simulink model "FinalSinScopes"  (R2023b)
settings: Solver=VariableStepAuto  StartTime=0.0  StopTime=10.0  RelTol=1e-3
values from neighbouring files (symbols this model uses):
  alfa_cu = 3.9E-3    (= 0.0039)    [Parametros.m]
  b_a = J_eq * n * omega_n    [MigracionPolosControladorExterno.m]    (also in Parametros.m = 1)
  b_eq = b_m + b_l/(r^2)    (= 2.19444444444e-05)    [Parametros.m]
  C_ts = 0.818    [Parametros.m]
  g = 9.80665    [Parametros.m]
  J_eq = J_m + J_l/(r^2)    [Parametros.m]
  k_l = m*l_cm + m_l(1)*l_l    [Parametros.m]
  K_sa = J_eq * n * omega_n^2    [MigracionPolosControladorExterno.m]    (also in Parametros.m = 1)
  K_sia = J_eq * omega_n^3    [MigracionPolosControladorExterno.m]    (also in Parametros.m = 1)
  Ke_int = 3.2768e10    (= 32768000000)    [Parametros.m]
  Ke_t = 6.4e3    (= 6400)    [Parametros.m]
  Ke_w = 1.024e7    (= 10240000)    [Parametros.m]
  L_d = 6.6E-3    (= 0.0066)    [Parametros.m]
  L_ls = 0.8E-3    (= 0.0008)    [Parametros.m]
  L_q = 5.8E-3    (= 0.0058)    [Parametros.m]
  lambda_m = 0.016    [Parametros.m]
  Mni_A = [0 -1; wn_mod^2 -2*zita_mod*wn_mod]    [Parametros.m]
  Mni_B = [1;0]    [Parametros.m]
  Mni_C = [0 1]    [Parametros.m]
  Mni_D = 0    [Parametros.m]
  P_p = 3    [Parametros.m]
  r = 120    [MigracionPolosControladorExterno.m]    (also in Parametros.m)
  R_tsamb = 146.7    [Parametros.m]
  Rs_ref = 1.02    [Parametros.m]
  Sni_A_iabc = [0 -1; wn_iabc^2 -2*wn_iabc*xi_iabc]    [Parametros.m]
  Sni_A_pos = [0 -1; wn_pos^2 -2*wn_pos*xi_pos]    [Parametros.m]
  Sni_A_T = -1/tau    (= -10)    [Parametros.m]
  Sni_B_iabc = [1; 0]    [Parametros.m]
  Sni_B_pos = [1; 0]    [Parametros.m]
  Sni_B_T = 1    [Parametros.m]
  Sni_C_iabc = [0 1]    [Parametros.m]
  Sni_C_pos = [0 1]    [Parametros.m]
  Sni_C_T = 1/tau    (= 10)    [Parametros.m]
  Sni_D_iabc = 0    [Parametros.m]
  Sni_D_pos = 0    [Parametros.m]
  Sni_D_T = 0    [Parametros.m]
  Tita_0 = 0    [Parametros.m]
  Ts = 1.25E-4    (= 0.000125)    [Parametros.m]
  Ts_0 = 20    [Parametros.m]
  Tsref = 20    [Parametros.m]
  V_slmax = 48    [Parametros.m]
settings Model: Creator=Home  LastModifiedBy=Home

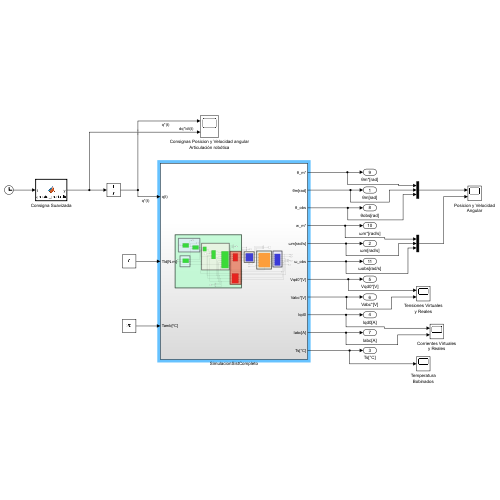
[thumbnail: Simulink's stored preview of the top-level diagram]
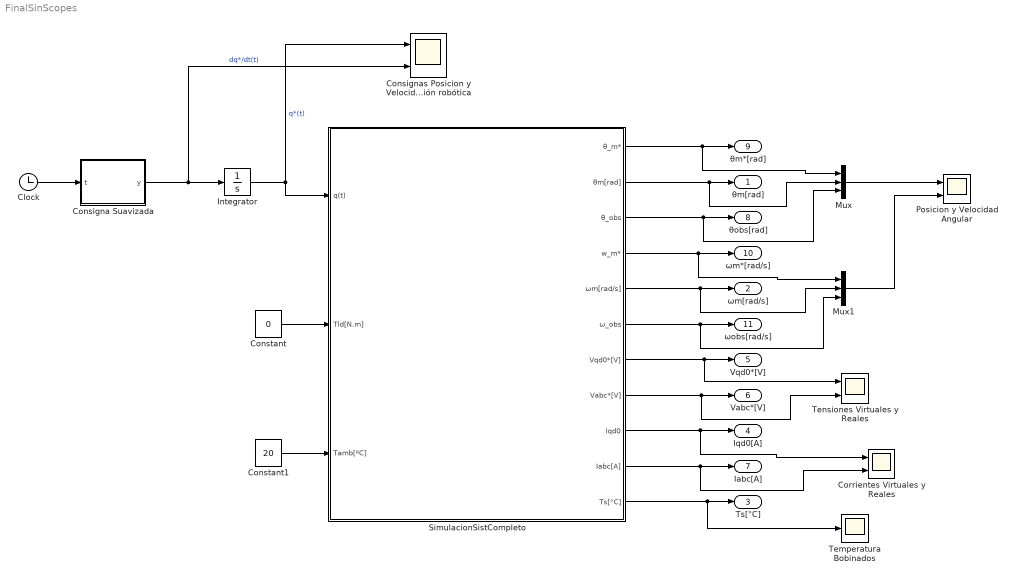
== system FinalSinScopes ==
  Clock : Clock
  Consigna Suavizada : MATLAB Function  TreatAsAtomicUnit=on
  Consignas Posicion y Velocidad angular Articulación robótica : Scope  NumInputPorts=2
  Constant : Constant  Value=0
  Constant1 : Constant  Value=20
  Corrientes Virtuales y Reales : Scope  NumInputPorts=2
  Integrator : Integrator
  Mux : Mux  Inputs=3
  Mux1 : Mux  Inputs=3
  Posicion y Velocidad Angular : Scope  NumInputPorts=2
  SimulacionSistCompleto : Subsystem
  Temperatura Bobinados : Scope
  Tensiones Virtuales y Reales : Scope  NumInputPorts=2
  θm[rad] : Outport
  ωm[rad/s] : Outport  Port=2
  Ts[°C] : Outport  Port=3
  Iqd0[A] : Outport  Port=4
  Vqd0*[V] : Outport  Port=5
  Vabc*[V] : Outport  Port=6
  Iabc[A] : Outport  Port=7
  θobs[rad] : Outport  Port=8
  θm*[rad] : Outport  Port=9
  ωm*[rad/s] : Outport  Port=10
  ωobs[rad/s] : Outport  Port=11
  wires:
  Integrator/1 -> Consignas Posicion y Velocidad angular Articulación robótica/1, SimulacionSistCompleto/1(q(t))  "q*(t)"
  SimulacionSistCompleto/2(θm[rad]) -> Mux/2, θm[rad]/1
  SimulacionSistCompleto/3(θ_obs) -> Mux/3, θobs[rad]/1
  Consigna Suavizada/1(y) -> Consignas Posicion y Velocidad angular Articulación robótica/2, Integrator/1  "dq*/dt(t)"
  Clock/1 -> Consigna Suavizada/1(t)
  Constant1/1 -> SimulacionSistCompleto/3(Tamb[ºC])
  SimulacionSistCompleto/1(θ_m*) -> Mux/1, θm*[rad]/1
  Constant/1 -> SimulacionSistCompleto/2(Tld[N.m])
  SimulacionSistCompleto/8(Vabc*[V]) -> Tensiones Virtuales y Reales/2, Vabc*[V]/1
  SimulacionSistCompleto/4(w_m*) -> Mux1/1, ωm*[rad/s]/1
  SimulacionSistCompleto/9(Iqd0) -> Corrientes Virtuales y Reales/1, Iqd0[A]/1
  SimulacionSistCompleto/5(ωm[rad/s]) -> Mux1/2, ωm[rad/s]/1
  SimulacionSistCompleto/10(Iabc[A]) -> Corrientes Virtuales y Reales/2, Iabc[A]/1
  SimulacionSistCompleto/11(Ts[°C]) -> Temperatura Bobinados/1, Ts[°C]/1
  SimulacionSistCompleto/7(Vqd0*[V]) -> Tensiones Virtuales y Reales/1, Vqd0*[V]/1
  SimulacionSistCompleto/6(ω_obs) -> Mux1/3, ωobs[rad/s]/1
  Mux/1 -> Posicion y Velocidad Angular/1
  Mux1/1 -> Posicion y Velocidad Angular/2

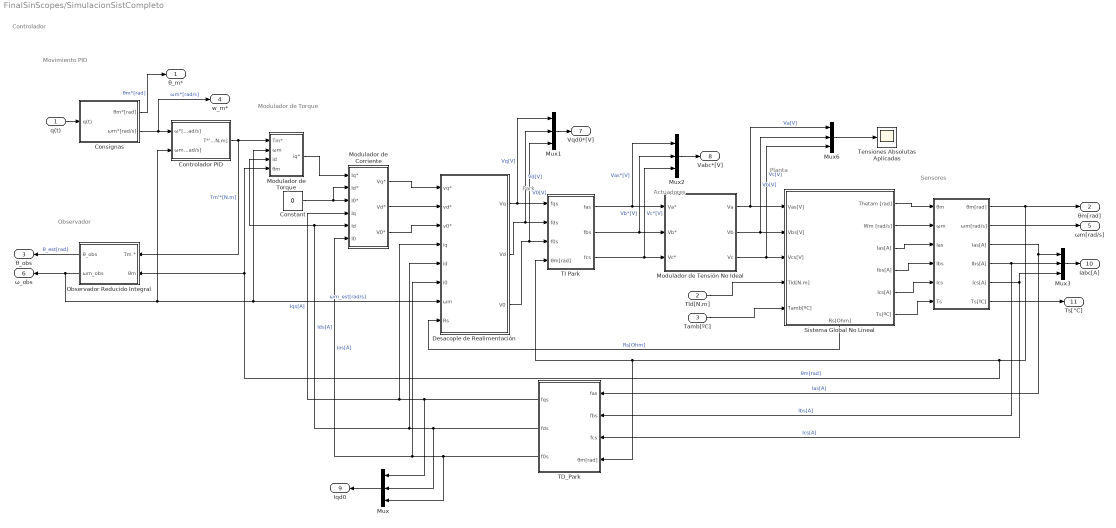
== system FinalSinScopes/SimulacionSistCompleto ==
  note: Sensores
  note: Park
  note: Observador
  note: Movimiento PID
  note: Modulador de Torque
  note: Controlador
  note: Actuadores
  note: Planta
  q(t) : Inport
  Tld[N.m] : Inport  Port=2
  Tamb[ºC] : Inport  Port=3
  " " : Subsystem
  Consignas : Subsystem
  Constant : Constant  Value=0
  Controlador PID : Subsystem
  Desacople de Realimentación : Subsystem
  Modulador de Corriente : Subsystem
  Modulador de Tensión No Ideal : Subsystem
  Modulador de Torque : Subsystem
  Mux{,1..3,6} (5 alike) : Mux  Inputs=3
  Observador Reducido Integral : Subsystem
  Sistema Global No Lineal : Subsystem
      settings: PortSchema="{\"entries\":[{\"content\":{\"sides\":[{\"content\":{\"connectorIds\":[\"In1\",\"In2\",\"In3\",\"In4\",\"In5\"]},\"type\":\"ConnectorPlacement.EquallySpacedRectSide\",\"uuid\":\"e69950d9-128a-479c-bb9c-058e9f1d4c4a\"},{\"content\":{\"connectorIds\":[\"Out1\",\"Out2\",\"Out3\",\"Out4\",\"Out5\",\"Out6\"],\"side\":\"RIGHT\"},\"type\":\"ConnectorPlacement.EquallySpacedRectSide\",\"uuid\":\"1754f544-d789-47dd-8fe5-32cce928f6e8\"},{\"content\":{\"side\":\"TOP\"},\"type\":\"ConnectorPlacement.EquallySpacedRectSide\",\"uuid\":\"429b420b-76ac-4d06-af5f-80d5ebf45ad3\"},{\"content\":{\"connectorIds\":[\"Out7\"],\"side\":\"BOTTOM\"},\"type\":\"ConnectorPlacement.EquallySpacedRectSide\",\"uuid\":\"85955431-78ef-4c8e-b012-5cf00baf8243\"}]},\"type\":\"ConnectorPlacement.EquallySpacedConnector\",\"uuid\":\"839c6553-6053-4832-bfe9-eda0736393b8\"}],\"packageUris\":[\"http://schema.mathworks.com/mf0/Connector/R2020b\"],\"version\":\"1.0\"}"
  TD_Park : Subsystem
  TI Park : Subsystem
  Tensiones Absolutas Aplicadas : Scope
  θ_m* : Outport
  θm[rad] : Outport  Port=2
  θ_obs : Outport  Port=3
  w_m* : Outport  Port=4
  ωm[rad/s] : Outport  Port=5
  ω_obs : Outport  Port=6
  Vqd0*[V] : Outport  Port=7
  Vabc*[V] : Outport  Port=8
  Iqd0 : Outport  Port=9
  Iabc[A] : Outport  Port=10
  Ts[°C] : Outport  Port=11
  wires:
  Consignas/2(ωm*[rad/s]) -> w_m*/1, Controlador PID/1(ω*[rad/s])  "ωm*[rad/s]"
  Modulador de Corriente/3(V0*) -> Desacople de Realimentación/3(v0*)
  Mux3/1 -> Iabc[A]/1
  TD_Park/2(fds) -> Modulador de Corriente/5(Id), Modulador de Torque/3(id), Desacople de Realimentación/5(id), Mux/2  "Ids[A]"
  TD_Park/1(fqs) -> Desacople de Realimentación/4(iq), Modulador de Corriente/4(Iq), Mux/1  "Iqs[A]"
  Modulador de Tensión No Ideal/3(Vc) -> Sistema Global No Lineal/3(Vcs[V]), Mux6/3  "Vc[V]"
  Modulador de Tensión No Ideal/1(Va) -> Sistema Global No Lineal/1(Vas[V]), Mux6/1  "Va[V]"
  Modulador de Torque/1(iq*) -> Modulador de Corriente/1(Iq*)
  TD_Park/3(f0s) -> Modulador de Corriente/6(I0), Desacople de Realimentación/6(i0), Mux/3  "Ios[A]"
  Modulador de Corriente/1(Vq*) -> Desacople de Realimentación/1(vq*)
  Desacople de Realimentación/2(Vd) -> Mux1/2, TI Park/2(fds)  "Vd[V]"
  Mux1/1 -> Vqd0*[V]/1
  Mux/1 -> Iqd0/1
  TI Park/1(fas) -> Modulador de Tensión No Ideal/1(Va*), Mux2/1  "Vas*[V]"
  TI Park/3(fcs) -> Modulador de Tensión No Ideal/3(Vc*), Mux2/3  "Vc*[V]"
  Tld[N.m]/1 -> Sistema Global No Lineal/4(Tld[N.m])
  Mux2/1 -> Vabc*[V]/1
  Tamb[ºC]/1 -> Sistema Global No Lineal/5(Tamb[ºC])
  Desacople de Realimentación/1(Vq) -> Mux1/1, TI Park/1(fqs)  "Vq[V]"
  Modulador de Corriente/2(Vd*) -> Desacople de Realimentación/2(vd*)
  Desacople de Realimentación/3(V0) -> Mux1/3, TI Park/3(f0s)  "V0[V]"
  q(t)/1 -> Consignas/1(q(t))
  Constant/1 -> Modulador de Corriente/3(I0*), Modulador de Corriente/2(Id*)
  TI Park/2(fbs) -> Modulador de Tensión No Ideal/2("Vb* "), Mux2/2  "Vb*[V]"
  Modulador de Tensión No Ideal/2(Vb) -> Sistema Global No Lineal/2(Vbs[V]), Mux6/2  "Vb[V]"
  Observador Reducido Integral/1(θ_obs) -> θ_obs/1  "θ_est[rad]"
  Controlador PID/1(T*'m[N.m]) -> Modulador de Torque/1(Tm*), Observador Reducido Integral/1(Tm *)  "Tm'*[N.m]"
  Observador Reducido Integral/2(ωm_obs) -> Desacople de Realimentación/7(ωm), Modulador de Torque/2(ωm), Controlador PID/2(ωm[rad/s]), ω_obs/1  "ωm_est[rad/s]"
  Consignas/1(θm*[rad]) -> θ_m*/1  "θm*[rad]"
  Sistema Global No Lineal/7(Rs[Ohm]) -> Desacople de Realimentación/8(Rs)  "Rs[Ohm]"
  Mux6/1 -> Tensiones Absolutas Aplicadas/1
  " "/3(Ias[A]) -> TD_Park/1(fas), Mux3/1  "Ias[A]"
  " "/5(Ics[A]) -> TD_Park/3(fcs), Mux3/3  "Ics[A]"
  " "/1(θm[rad]) -> θm[rad]/1, Observador Reducido Integral/2(θm), Modulador de Torque/4(θm), TD_Park/4(θm[rad]), TI Park/4(θm[rad])  "θm[rad]"
  " "/4(Ibs[A]) -> TD_Park/2(fbs), Mux3/2  "Ibs[A]"
  Sistema Global No Lineal/1(Thetam [rad]) -> " "/1(θm)
  Sistema Global No Lineal/2(Wm [rad/s]) -> " "/2(ωm)
  Sistema Global No Lineal/3(Ias[A]) -> " "/3(Ias)
  Sistema Global No Lineal/4(Ibs[A]) -> " "/4(Ibs)
  Sistema Global No Lineal/5(Ics[A]) -> " "/5(Ics)
  Sistema Global No Lineal/6(Ts[ºC]) -> " "/6(Ts)
  " "/2(ωm[rad/s]) -> ωm[rad/s]/1
  " "/6(Ts[ºC]) -> Ts[°C]/1

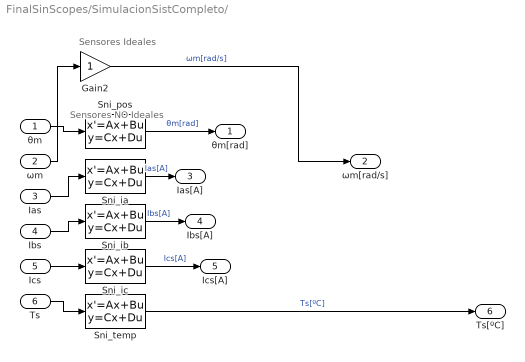
== system FinalSinScopes/SimulacionSistCompleto/  ==
  note: Sensores NO Ideales
  note: Sensores Ideales
  θm : Inport
  ωm : Inport  Port=2
  Ias : Inport  Port=3
  Ibs : Inport  Port=4
  Ics : Inport  Port=5
  Ts : Inport  Port=6
  Gain2 : Gain
  Sni_ia : StateSpace  A=Sni_A_iabc  B=Sni_B_iabc  C=Sni_C_iabc  D=Sni_D_iabc  InitialCondition=0
  Sni_ib : StateSpace  A=Sni_A_iabc  B=Sni_B_iabc  C=Sni_C_iabc  D=Sni_D_iabc  InitialCondition=0
  Sni_ic : StateSpace  A=Sni_A_iabc  B=Sni_B_iabc  C=Sni_C_iabc  D=Sni_D_iabc  InitialCondition=0
  Sni_pos : StateSpace  A=Sni_A_pos  B=Sni_B_pos  C=Sni_C_pos  D=Sni_D_pos  InitialCondition=0
  Sni_temp : StateSpace  A=Sni_A_T  B=Sni_B_T  C=Sni_C_T  D=Sni_D_T  InitialCondition=0
  θm[rad] : Outport
  ωm[rad/s] : Outport  Port=2
  Ias[A] : Outport  Port=3
  Ibs[A] : Outport  Port=4
  Ics[A] : Outport  Port=5
  Ts[ºC] : Outport  Port=6
  wires:
  Ics/1 -> Sni_ic/1
  Gain2/1 -> ωm[rad/s]/1  "ωm[rad/s]"
  Ibs/1 -> Sni_ib/1
  θm/1 -> Sni_pos/1
  Ts/1 -> Sni_temp/1
  Ias/1 -> Sni_ia/1
  Sni_temp/1 -> Ts[ºC]/1  "Ts[ºC]"
  Sni_pos/1 -> θm[rad]/1  "θm[rad]"
  ωm/1 -> Gain2/1
  Sni_ic/1 -> Ics[A]/1  "Ics[A]"
  Sni_ia/1 -> Ias[A]/1  "Ias[A]"
  Sni_ib/1 -> Ibs[A]/1  "Ibs[A]"

== system FinalSinScopes/SimulacionSistCompleto/Consignas ==
  q(t) : Inport
  Derivative : Derivative
  Gain : Gain  Gain=r
  θm*[rad] : Outport
  ωm*[rad/s] : Outport  Port=2
  wires:
  Derivative/1 -> ωm*[rad/s]/1
  Gain/1 -> θm*[rad]/1, Derivative/1
  q(t)/1 -> Gain/1

== system FinalSinScopes/SimulacionSistCompleto/Controlador PID ==
  ω*[rad/s] : Inport
  ωm[rad/s] : Inport  Port=2
  Gain : Gain  Gain=b_a
  Gain1 : Gain  Gain=K_sia
  Gain2 : Gain  Gain=K_sa
  Integracion Tustin : Subsystem
  Integracion Tustin1 : Subsystem
  Sum : Sum  Inputs=|+-
  Sum1 : Sum  Inputs=+++
  Zero-Order Hold : ZeroOrderHold  SampleTime=Ts
  Zero-Order Hold1 : ZeroOrderHold  SampleTime=Ts
  T*'m[N.m] : Outport
  wires:
  Sum1/1 -> Zero-Order Hold1/1
  Integracion Tustin1/1(y[k]) -> Gain1/1
  ω*[rad/s]/1 -> Sum/1
  Zero-Order Hold/1 -> Integracion Tustin/1(x[k]), Gain/1  "Ew"
  Gain2/1 -> Sum1/2
  Integracion Tustin/1(y[k]) -> Integracion Tustin1/1(x[k]), Gain2/1  "Eθ"
  ωm[rad/s]/1 -> Sum/2
  Gain/1 -> Sum1/3
  Gain1/1 -> Sum1/1
  Sum/1 -> Zero-Order Hold/1  "Ew"
  Zero-Order Hold1/1 -> T*'m[N.m]/1

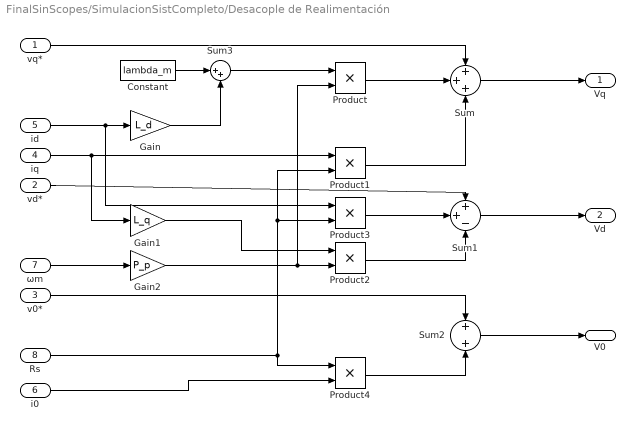
== system FinalSinScopes/SimulacionSistCompleto/Desacople de Realimentación ==
  vq* : Inport
  vd* : Inport  Port=2
  v0* : Inport  Port=3
  iq : Inport  Port=4
  id : Inport  Port=5
  i0 : Inport  Port=6
  ωm : Inport  Port=7
  Rs : Inport  Port=8
  Constant : Constant  Value=lambda_m
  Gain : Gain  Gain=L_d
  Gain1 : Gain  Gain=L_q
  Gain2 : Gain  Gain=P_p
  Product{,1..4} (5 alike) : Product
  Sum : Sum  Inputs=+++
  Sum1 : Sum  Inputs=++-
  Sum2 : Sum  Inputs=+|+
  Sum3 : Sum  Inputs=|++
  Vq : Outport
  Vd : Outport  Port=2
  V0 : Outport  Port=3
  wires:
  ωm/1 -> Gain2/1
  Sum/1 -> Vq/1
  Rs/1 -> Product4/1, Product1/2, Product3/2
  Gain/1 -> Sum3/2
  Product/1 -> Sum/2
  Sum2/1 -> V0/1
  Product4/1 -> Sum2/2
  Sum3/1 -> Product/1
  id/1 -> Product3/1, Gain/1
  vq*/1 -> Sum/1
  i0/1 -> Product4/2
  iq/1 -> Product1/1, Gain1/1
  Product2/1 -> Sum1/3
  Constant/1 -> Sum3/1
  v0*/1 -> Sum2/1
  Product1/1 -> Sum/3
  Gain2/1 -> Product/2, Product2/2
  vd*/1 -> Sum1/1
  Gain1/1 -> Product2/1
  Sum1/1 -> Vd/1
  Product3/1 -> Sum1/2

== system FinalSinScopes/SimulacionSistCompleto/Modulador de Corriente ==
  Iq* : Inport
  Id* : Inport  Port=2
  I0* : Inport  Port=3
  Iq : Inport  Port=4
  Id : Inport  Port=5
  I0 : Inport  Port=6
  Gain : Gain  Gain=5000*L_q
  Gain1 : Gain  Gain=5000*L_d
  Gain2 : Gain  Gain=5000*L_ls
  Sum : Sum  Inputs=|+-
  Sum1 : Sum  Inputs=|+-
  Sum2 : Sum  Inputs=|+-
  Vq* : Outport
  Vd* : Outport  Port=2
  V0* : Outport  Port=3
  wires:
  Gain2/1 -> V0*/1
  Sum/1 -> Gain/1
  Sum1/1 -> Gain1/1
  Gain/1 -> Vq*/1
  Iq/1 -> Sum/2
  I0*/1 -> Sum2/1
  Iq*/1 -> Sum/1
  Id/1 -> Sum1/2
  Sum2/1 -> Gain2/1
  Id*/1 -> Sum1/1
  Gain1/1 -> Vd*/1
  I0/1 -> Sum2/2

== system FinalSinScopes/SimulacionSistCompleto/Modulador de Tensión No Ideal ==
  Va* : Inport
  "Vb* " : Inport  Port=2
  Vc* : Inport  Port=3
  Saturation : Saturate  UpperLimit=sqrt(2/3)*V_slmax  LowerLimit=-sqrt(2/3)*V_slmax
  Saturation1 : Saturate  UpperLimit=sqrt(2/3)*V_slmax  LowerLimit=-sqrt(2/3)*V_slmax
  Saturation2 : Saturate  UpperLimit=sqrt(2/3)*V_slmax  LowerLimit=-sqrt(2/3)*V_slmax
  State-Space : StateSpace  A=Mni_A  B=Mni_B  C=Mni_C  D=Mni_D  InitialCondition=0
  State-Space1 : StateSpace  A=Mni_A  B=Mni_B  C=Mni_C  D=Mni_D  InitialCondition=0
  State-Space2 : StateSpace  A=Mni_A  B=Mni_B  C=Mni_C  D=Mni_D  InitialCondition=0
  Va : Outport
  Vb : Outport  Port=2
  Vc : Outport  Port=3
  wires:
  Vc*/1 -> State-Space2/1
  "Vb* "/1 -> State-Space1/1
  State-Space/1 -> Saturation/1
  Va*/1 -> State-Space/1
  State-Space1/1 -> Saturation1/1
  State-Space2/1 -> Saturation2/1
  Saturation/1 -> Va/1
  Saturation1/1 -> Vb/1
  Saturation2/1 -> Vc/1

== system FinalSinScopes/SimulacionSistCompleto/Modulador de Torque ==
  Tm* : Inport
  ωm : Inport  Port=2
  id : Inport  Port=3
  θm : Inport  Port=4
  Constant : Constant  Value=L_d
  Constant1 : Constant  Value=L_q
  Constant2 : Constant  Value=lambda_m
  Divide : Product  Inputs=*/
  Gain : Gain  Gain=b_eq
  Gain1 : Gain  Gain=3/2*P_p
  Gain2 : Gain  Gain=1/r
  Gain3 : Gain  Gain=k_l*g/r
  Product : Product
  Sin : Trigonometry
  Sum : Sum  Inputs=+++
  Sum1 : Sum  Inputs=|+-
  Sum2 : Sum  Inputs=|++
  iq* : Outport
  wires:
  Constant2/1 -> Sum2/2
  ωm/1 -> Gain/1
  Sum1/1 -> Product/2
  Gain3/1 -> Sum/1
  θm/1 -> Gain2/1  "θm"
  Sum2/1 -> Gain1/1
  Constant/1 -> Sum1/1
  Gain1/1 -> Divide/2
  Divide/1 -> iq*/1
  Product/1 -> Sum2/1
  Gain/1 -> Sum/3
  Constant1/1 -> Sum1/2
  Sin/1 -> Gain3/1
  Gain2/1 -> Sin/1
  Sum/1 -> Divide/1
  id/1 -> Product/1
  Tm*/1 -> Sum/2

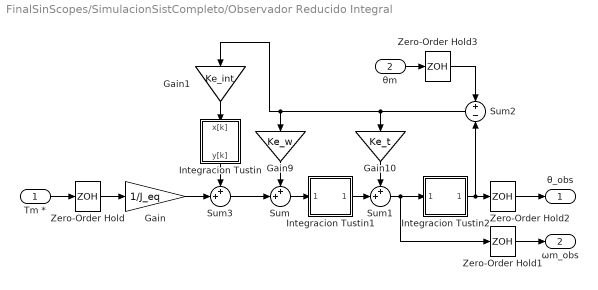
== system FinalSinScopes/SimulacionSistCompleto/Observador Reducido Integral ==
  Tm * : Inport
  θm : Inport  Port=2
  Gain : Gain  Gain=1/J_eq
  Gain1 : Gain  Gain=Ke_int
  Gain10 : Gain  Gain=Ke_t
  Gain9 : Gain  Gain=Ke_w
  Integracion Tustin : Subsystem
  Integracion Tustin1 : Subsystem
  Integracion Tustin2 : Subsystem
  Sum : Sum  Inputs=++|
  Sum1 : Sum  Inputs=++|
  Sum2 : Sum  Inputs=+|-
  Sum3 : Sum  Inputs=++|
  Zero-Order Hold{,1..3} (4 alike) : ZeroOrderHold  SampleTime=-1
  θ_obs : Outport
  ωm_obs : Outport  Port=2
  wires:
  Gain10/1 -> Sum1/1
  Sum2/1 -> Gain1/1, Gain9/1, Gain10/1
  Integracion Tustin2/1(y[k]) -> Zero-Order Hold2/1, Sum2/2
  Tm */1 -> Zero-Order Hold/1
  θm/1 -> Zero-Order Hold3/1
  Sum1/1 -> Integracion Tustin2/1(x[k]), Zero-Order Hold1/1
  Integracion Tustin1/1(y[k]) -> Sum1/2
  Sum/1 -> Integracion Tustin1/1(x[k])
  Gain/1 -> Sum3/2
  Gain9/1 -> Sum/1
  Sum3/1 -> Sum/2
  Gain1/1 -> Integracion Tustin/1(x[k])
  Integracion Tustin/1(y[k]) -> Sum3/1
  Zero-Order Hold/1 -> Gain/1
  Zero-Order Hold1/1 -> ωm_obs/1
  Zero-Order Hold2/1 -> θ_obs/1
  Zero-Order Hold3/1 -> Sum2/1

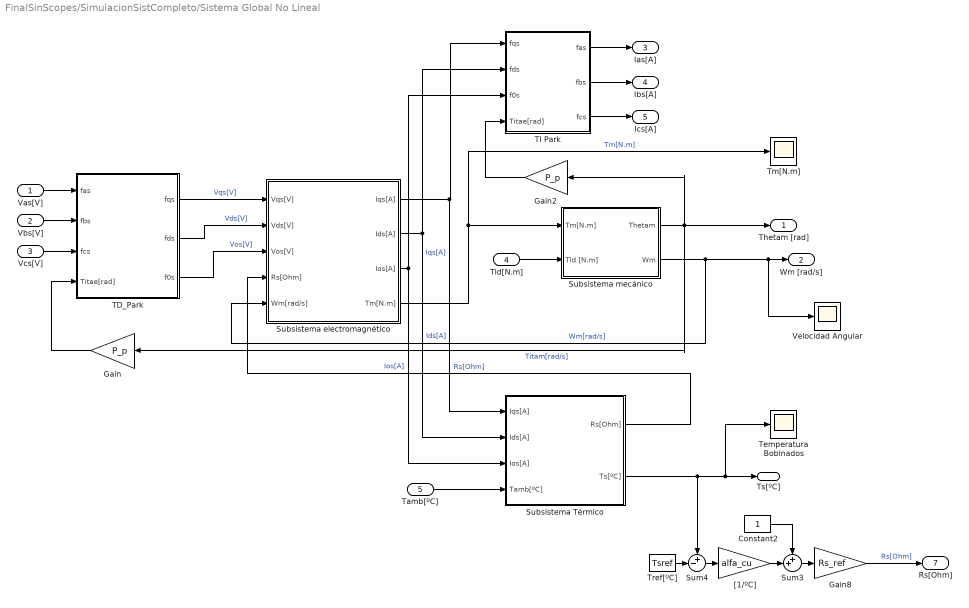
== system FinalSinScopes/SimulacionSistCompleto/Sistema Global No Lineal ==
  Vas[V] : Inport
  Vbs[V] : Inport  Port=2
  Vcs[V] : Inport  Port=3
  Tld[N.m] : Inport  Port=4
  Tamb[ºC] : Inport  Port=5
  Constant2 : Constant
  Gain : Gain  Gain=P_p
  Gain2 : Gain  Gain=P_p
  Gain8 : Gain  Gain=Rs_ref
  Subsistema Térmico : Subsystem
  Subsistema electromagnético : Subsystem
  Subsistema mecánico : Subsystem
  Sum3 : Sum  Inputs=++|
  Sum4 : Sum  Inputs=+-|
  TD_Park : Subsystem
  TI Park : Subsystem
  Temperatura Bobinados : Scope
  Tm[N.m] : Scope
  Tref[ºC] : Constant  Value=Tsref
  Velocidad Angular : Scope
  "[1/ºC]" : Gain  Gain=alfa_cu
  Thetam [rad] : Outport
  Wm [rad/s] : Outport  Port=2
  Ias[A] : Outport  Port=3
  Ibs[A] : Outport  Port=4
  Ics[A] : Outport  Port=5
  Ts[ºC] : Outport  Port=6
  Rs[Ohm] : Outport  Port=7
  wires:
  Subsistema electromagnético/3(Ios[A]) -> Subsistema Térmico/3(Ios[A]), TI Park/3(f0s)  "Ios[A]"
  Subsistema mecánico/2(Wm) -> Velocidad Angular/1, Wm [rad/s]/1, Subsistema electromagnético/5(Wm[rad/s])  "Wm[rad/s]"
  TD_Park/3(f0s) -> Subsistema electromagnético/3(Vos[V])  "Vos[V]"
  Gain/1 -> TD_Park/4(Titae[rad])
  Subsistema Térmico/1(Rs[Ohm]) -> Subsistema electromagnético/4(Rs[Ohm])  "Rs[Ohm]"
  TD_Park/1(fqs) -> Subsistema electromagnético/1(Vqs[V])  "Vqs[V]"
  Vbs[V]/1 -> TD_Park/2(fbs)
  Vcs[V]/1 -> TD_Park/3(fcs)
  Subsistema electromagnético/1(Iqs[A]) -> Subsistema Térmico/1(Iqs[A]), TI Park/1(fqs)  "Iqs[A]"
  Subsistema electromagnético/4(Tm[N.m]) -> Tm[N.m]/1, Subsistema mecánico/1(Tm[N.m])  "Tm[N.m]"
  Subsistema mecánico/1(Thetam) -> Thetam [rad]/1, Gain2/1, Gain/1  "Titam[rad/s]"
  Tamb[ºC]/1 -> Subsistema Térmico/4(Tamb[ºC])
  Vas[V]/1 -> TD_Park/1(fas)
  TD_Park/2(fds) -> Subsistema electromagnético/2(Vds[V])  "Vds[V]"
  TI Park/2(fbs) -> Ibs[A]/1
  Subsistema electromagnético/2(Ids[A]) -> TI Park/2(fds), Subsistema Térmico/2(Ids[A])  "Ids[A]"
  Gain2/1 -> TI Park/4(Titae[rad])
  TI Park/1(fas) -> Ias[A]/1
  Subsistema Térmico/2(Ts[ºC]) -> Sum4/1, Temperatura Bobinados/1, Ts[ºC]/1
  Tld[N.m]/1 -> Subsistema mecánico/2(Tld [N.m])
  TI Park/3(fcs) -> Ics[A]/1
  "[1/ºC]"/1 -> Sum3/2
  Sum3/1 -> Gain8/1
  Tref[ºC]/1 -> Sum4/2
  Constant2/1 -> Sum3/1
  Sum4/1 -> "[1/ºC]"/1
  Gain8/1 -> Rs[Ohm]/1  "Rs[Ohm]"

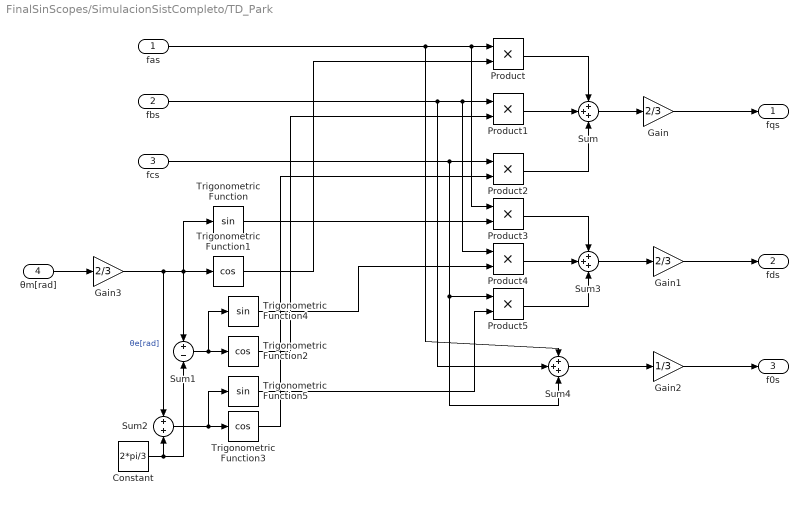
== system FinalSinScopes/SimulacionSistCompleto/TD_Park ==
  fas : Inport
  fbs : Inport  Port=2
  fcs : Inport  Port=3
  θm[rad] : Inport  Port=4
  Constant : Constant  Value=2*pi/3
  Gain : Gain  Gain=2/3
  Gain1 : Gain  Gain=2/3
  Gain2 : Gain  Gain=1/3
  Gain3 : Gain  Gain=2/3
  Product{,1..5} (6 alike) : Product
  Sum : Sum  Inputs=+++
  Sum1 : Sum  Inputs=+-
  Sum2 : Sum
  Sum3 : Sum  Inputs=+++
  Sum4 : Sum  Inputs=+++
  Trigonometric Function : Trigonometry
  Trigonometric Function1 : Trigonometry  Operator=cos
  Trigonometric Function2 : Trigonometry  Operator=cos
  Trigonometric Function3 : Trigonometry  Operator=cos
  Trigonometric Function4 : Trigonometry
  Trigonometric Function5 : Trigonometry
  fqs : Outport
  fds : Outport  Port=2
  f0s : Outport  Port=3
  wires:
  fas/1 -> Sum4/1, Product3/1, Product/1
  Trigonometric Function3/1 -> Product2/2
  Sum1/1 -> Trigonometric Function4/1, Trigonometric Function2/1
  Constant/1 -> Sum2/2, Sum1/2
  Trigonometric Function1/1 -> Product/2
  fcs/1 -> Product5/1, Sum4/3, Product2/1
  Product5/1 -> Sum3/3
  Product/1 -> Sum/1
  Product3/1 -> Sum3/1
  Product1/1 -> Sum/2
  Trigonometric Function/1 -> Product3/2
  Sum2/1 -> Trigonometric Function5/1, Trigonometric Function3/1
  Trigonometric Function5/1 -> Product5/2
  Sum4/1 -> Gain2/1
  fbs/1 -> Sum4/2, Product4/1, Product1/1
  Product2/1 -> Sum/3
  Gain/1 -> fqs/1
  Trigonometric Function4/1 -> Product4/2
  Product4/1 -> Sum3/2
  Trigonometric Function2/1 -> Product1/2
  Gain2/1 -> f0s/1
  Sum/1 -> Gain/1
  Gain1/1 -> fds/1
  Sum3/1 -> Gain1/1
  θm[rad]/1 -> Gain3/1
  Gain3/1 -> Sum2/1, Trigonometric Function/1, Sum1/1, Trigonometric Function1/1  "θe[rad]"

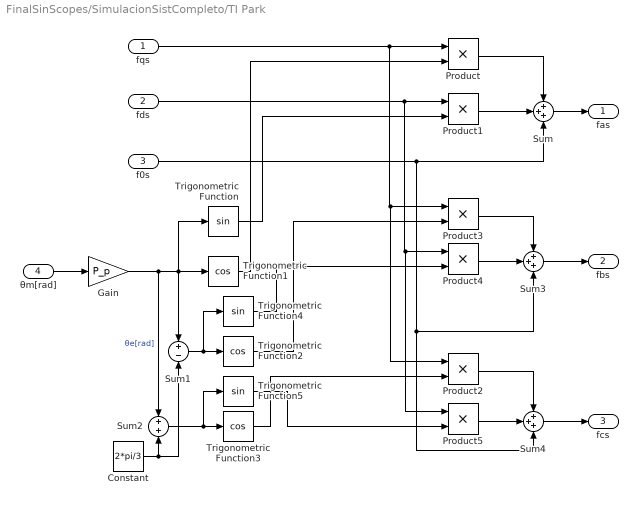
== system FinalSinScopes/SimulacionSistCompleto/TI Park ==
  fqs : Inport
  fds : Inport  Port=2
  f0s : Inport  Port=3
  θm[rad] : Inport  Port=4
  Constant : Constant  Value=2*pi/3
  Gain : Gain  Gain=P_p
  Product{,1..5} (6 alike) : Product
  Sum : Sum  Inputs=+++
  Sum1 : Sum  Inputs=+-
  Sum2 : Sum
  Sum3 : Sum  Inputs=+++
  Sum4 : Sum  Inputs=+++
  Trigonometric Function : Trigonometry
  Trigonometric Function1 : Trigonometry  Operator=cos
  Trigonometric Function2 : Trigonometry  Operator=cos
  Trigonometric Function3 : Trigonometry  Operator=cos
  Trigonometric Function4 : Trigonometry
  Trigonometric Function5 : Trigonometry
  fas : Outport
  fbs : Outport  Port=2
  fcs : Outport  Port=3
  wires:
  Constant/1 -> Sum2/2, Sum1/2
  Product1/1 -> Sum/2
  Trigonometric Function2/1 -> Product3/2
  Trigonometric Function5/1 -> Product5/2
  fds/1 -> Product1/1, Product5/1, Product4/1
  f0s/1 -> Sum/3, Sum3/3, Sum4/3
  Product3/1 -> Sum3/1
  fqs/1 -> Product/1, Product2/1, Product3/1
  Product2/1 -> Sum4/1
  Trigonometric Function1/1 -> Product/2
  Product/1 -> Sum/1
  Sum2/1 -> Trigonometric Function5/1, Trigonometric Function3/1
  Sum1/1 -> Trigonometric Function4/1, Trigonometric Function2/1
  Trigonometric Function/1 -> Product1/2
  Product4/1 -> Sum3/2
  Sum/1 -> fas/1
  Trigonometric Function3/1 -> Product2/2
  Product5/1 -> Sum4/2
  Trigonometric Function4/1 -> Product4/2
  Sum3/1 -> fbs/1
  Sum4/1 -> fcs/1
  θm[rad]/1 -> Gain/1
  Gain/1 -> Sum2/1, Trigonometric Function/1, Sum1/1, Trigonometric Function1/1  "θe[rad]"

== system FinalSinScopes/SimulacionSistCompleto/Controlador PID/Integracion Tustin ==
  x[k] : Inport
  Delay : Delay  DelayLength=1
  Delay1 : Delay  DelayLength=1
  Gain3 : Gain  Gain=Ts/2
  Sum2 : Sum  Inputs=|++
  Sum3 : Sum  Inputs=|++
  y[k] : Outport
  wires:
  x[k]/1 -> Delay/1, Sum3/1
  Sum2/1 -> y[k]/1, Delay1/1
  Delay1/1 -> Sum2/2
  Sum3/1 -> Gain3/1
  Delay/1 -> Sum3/2
  Gain3/1 -> Sum2/1

== system FinalSinScopes/SimulacionSistCompleto/Controlador PID/Integracion Tustin1 ==
  x[k] : Inport
  Delay : Delay  DelayLength=1
  Delay1 : Delay  DelayLength=1
  Gain3 : Gain  Gain=Ts/2
  Sum2 : Sum  Inputs=|++
  Sum3 : Sum  Inputs=|++
  y[k] : Outport
  wires:
  x[k]/1 -> Delay/1, Sum3/1
  Sum2/1 -> y[k]/1, Delay1/1
  Delay1/1 -> Sum2/2
  Sum3/1 -> Gain3/1
  Delay/1 -> Sum3/2
  Gain3/1 -> Sum2/1

== system FinalSinScopes/SimulacionSistCompleto/Observador Reducido Integral/Integracion Tustin ==
  x[k] : Inport
  Delay : Delay  DelayLength=1
  Delay1 : Delay  DelayLength=1
  Gain3 : Gain  Gain=Ts/2
  Sum2 : Sum  Inputs=|++
  Sum3 : Sum  Inputs=|++
  y[k] : Outport
  wires:
  x[k]/1 -> Delay/1, Sum3/1
  Sum2/1 -> y[k]/1, Delay1/1
  Delay1/1 -> Sum2/2
  Sum3/1 -> Gain3/1
  Delay/1 -> Sum3/2
  Gain3/1 -> Sum2/1

== system FinalSinScopes/SimulacionSistCompleto/Observador Reducido Integral/Integracion Tustin1 ==
  x[k] : Inport
  Delay : Delay  DelayLength=1
  Delay1 : Delay  DelayLength=1
  Gain3 : Gain  Gain=Ts/2
  Sum2 : Sum  Inputs=|++
  Sum3 : Sum  Inputs=|++
  y[k] : Outport
  wires:
  x[k]/1 -> Delay/1, Sum3/1
  Sum2/1 -> y[k]/1, Delay1/1
  Delay1/1 -> Sum2/2
  Sum3/1 -> Gain3/1
  Delay/1 -> Sum3/2
  Gain3/1 -> Sum2/1

== system FinalSinScopes/SimulacionSistCompleto/Observador Reducido Integral/Integracion Tustin2 ==
  x[k] : Inport
  Delay : Delay  DelayLength=1
  Delay1 : Delay  DelayLength=1
  Gain3 : Gain  Gain=Ts/2
  Sum2 : Sum  Inputs=|++
  Sum3 : Sum  Inputs=|++
  y[k] : Outport
  wires:
  x[k]/1 -> Delay/1, Sum3/1
  Sum2/1 -> y[k]/1, Delay1/1
  Delay1/1 -> Sum2/2
  Sum3/1 -> Gain3/1
  Delay/1 -> Sum3/2
  Gain3/1 -> Sum2/1

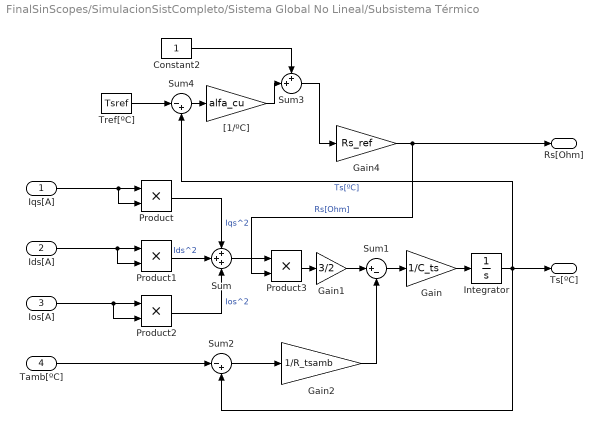
== system FinalSinScopes/SimulacionSistCompleto/Sistema Global No Lineal/Subsistema Térmico ==
  Iqs[A] : Inport
  Ids[A] : Inport  Port=2
  Ios[A] : Inport  Port=3
  Tamb[ºC] : Inport  Port=4
  Constant2 : Constant
  Gain : Gain  Gain=1/C_ts
  Gain1 : Gain  Gain=3/2
  Gain2 : Gain  Gain=1/R_tsamb
  Gain4 : Gain  Gain=Rs_ref
  Integrator : Integrator  InitialCondition=Ts_0
  Product{,1..3} (4 alike) : Product
  Sum : Sum  Inputs=+++
  Sum1 : Sum  Inputs=|+-
  Sum2 : Sum  Inputs=|-+
  Sum3 : Sum  Inputs=++|
  Sum4 : Sum  Inputs=|-+
  Tref[ºC] : Constant  Value=Tsref
  "[1/ºC]" : Gain  Gain=alfa_cu
  Rs[Ohm] : Outport
  Ts[ºC] : Outport  Port=2
  wires:
  Sum3/1 -> Gain4/1
  Gain/1 -> Integrator/1
  Product1/1 -> Sum/2  "Ids^2"
  Product/1 -> Sum/1  "Iqs^2"
  Sum/1 -> Product3/1
  Iqs[A]/1 -> Product/2, Product/1
  Ids[A]/1 -> Product1/2, Product1/1
  Product2/1 -> Sum/3  "Ios^2"
  Sum4/1 -> "[1/ºC]"/1
  Tamb[ºC]/1 -> Sum2/1
  Sum1/1 -> Gain/1
  Sum2/1 -> Gain2/1
  Gain4/1 -> Rs[Ohm]/1, Product3/2  "Rs[Ohm]"
  Gain1/1 -> Sum1/1
  Ios[A]/1 -> Product2/2, Product2/1
  Constant2/1 -> Sum3/1
  Tref[ºC]/1 -> Sum4/1
  Product3/1 -> Gain1/1
  "[1/ºC]"/1 -> Sum3/2
  Gain2/1 -> Sum1/2
  Integrator/1 -> Ts[ºC]/1, Sum2/2, Sum4/2  "Ts[ºC]"

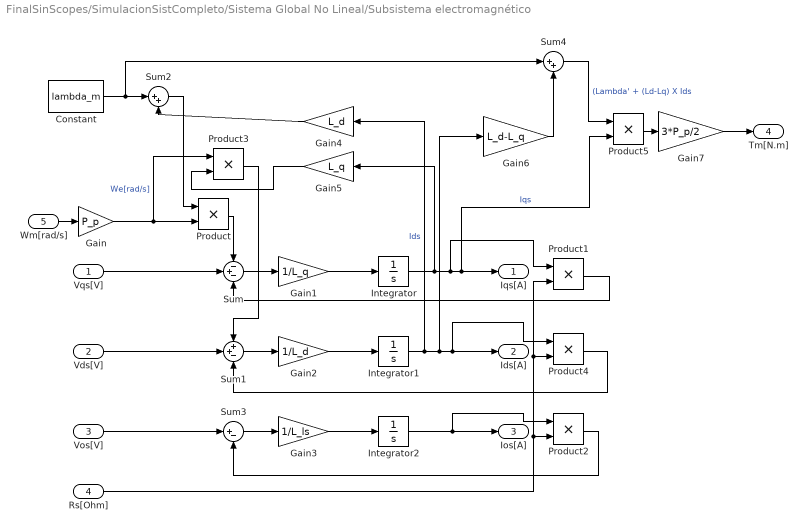
== system FinalSinScopes/SimulacionSistCompleto/Sistema Global No Lineal/Subsistema electromagnético ==
  Vqs[V] : Inport
  Vds[V] : Inport  Port=2
  Vos[V] : Inport  Port=3
  Rs[Ohm] : Inport  Port=4
  Wm[rad/s] : Inport  Port=5
  Constant : Constant  Value=lambda_m
  Gain : Gain  Gain=P_p
  Gain1 : Gain  Gain=1/L_q
  Gain2 : Gain  Gain=1/L_d
  Gain3 : Gain  Gain=1/L_ls
  Gain4 : Gain  Gain=L_d
  Gain5 : Gain  Gain=L_q
  Gain6 : Gain  Gain=L_d-L_q
  Gain7 : Gain  Gain=3*P_p/2
  Integrator : Integrator
  Integrator1 : Integrator  InitialCondition=-0.5
  Integrator2 : Integrator
  Product{,1..5} (6 alike) : Product
  Sum : Sum  Inputs=-+-
  Sum1 : Sum  Inputs=++-
  Sum2 : Sum  Inputs=|++
  Sum3 : Sum  Inputs=|+-
  Sum4 : Sum  Inputs=|++
  Iqs[A] : Outport
  Ids[A] : Outport  Port=2
  Ios[A] : Outport  Port=3
  Tm[N.m] : Outport  Port=4
  wires:
  Product3/1 -> Sum1/1
  Gain5/1 -> Product3/2
  Vos[V]/1 -> Sum3/1
  Sum1/1 -> Gain2/1
  Integrator/1 -> Gain5/1, Product1/1, Iqs[A]/1, Product5/2  "Iqs"
  Integrator2/1 -> Ios[A]/1, Product2/1
  Rs[Ohm]/1 -> Product4/2, Product1/2, Product2/2
  Product1/1 -> Sum/3
  Sum/1 -> Gain1/1
  Sum4/1 -> Product5/1  "(Lambda' + (Ld-Lq) X Ids"
  Integrator1/1 -> Gain6/1, Ids[A]/1, Product4/1, Gain4/1  "Ids"
  Gain/1 -> Product/2, Product3/1  "We[rad/s]"
  Sum3/1 -> Gain3/1
  Gain6/1 -> Sum4/2
  Wm[rad/s]/1 -> Gain/1
  Gain7/1 -> Tm[N.m]/1
  Product5/1 -> Gain7/1
  Vqs[V]/1 -> Sum/2
  Gain2/1 -> Integrator1/1
  Product/1 -> Sum/1
  Constant/1 -> Sum4/1, Sum2/1
  Sum2/1 -> Product/1
  Vds[V]/1 -> Sum1/2
  Gain4/1 -> Sum2/2
  Product4/1 -> Sum1/3
  Product2/1 -> Sum3/2
  Gain1/1 -> Integrator/1
  Gain3/1 -> Integrator2/1

== system FinalSinScopes/SimulacionSistCompleto/Sistema Global No Lineal/Subsistema mecánico ==
  note: beq [N.m/{rad/s}]
  note: 1/Jeq [kg.m^2]
  Tm[N.m] : Inport
  Tld [N.m] : Inport  Port=2
  Gain : Gain  Gain=1/J_eq
  Gain1 : Gain  Gain=b_eq
  Gain2 : Gain  Gain=g*k_l/r
  Gain3 : Gain  Gain=1/r
  Gain4 : Gain  Gain=1/r
  Integrator : Integrator
  Integrator1 : Integrator  InitialCondition=Tita_0
  Perturbacion TL : Scope
  Sum1 : Sum  Inputs=-+-
  Sum2 : Sum  Inputs=|++
  TorqueEq : Scope
  TorqueFriccion : Scope
  Trigonometric Function : Trigonometry
  XY Graph : Record  FileSettingsInternal="{\"entries\":[{\"content\":{\"excelSettings\":{\"content\":{},\"type\":\"Streamout.ExcelSettings\"}},\"type\":\"Streamout.FileSettingStorage\",\"uuid\":\"\"}],\"packageUris\":[\"http:\\/\\/schema.mathworks.com\\/mf0\\/streamout_blocks\\/R2020a\"],\"version\":\"1.0\"}"  Layout=[1 1]  SignalsInternal="{\"entries\":[{\"content\":{\"signals\":[{\"content\":{\"blockPath\":[],\"dimensions\":[1],\"domain\":\"\",\"lineColor\":\"#ff6929\",\"port\":1,\"signalID\":14343,\"signalName\":\"Wm[rad\\/s]\"},\"type\":\"RecordBlkView.Signal\",\"uuid\":\"\"},{\"content\":{\"blockPath\":[],\"dimensions\":[1],\"domain\":\"\",\"lineColor\":\"#b746ff\",\"port\":2,\"signalID\":14346,\"signalName\":\"Tm[N.m]\"},\"type\":\"RecordBlkView.Signal\",\"uuid\":\"\"}]},\"type\":\"RecordBlkView.InputSignals\",\"uuid\":\"\"}],\"packageUris\":[\"http:\\/\\/schema.mathworks.com\\/mf0\\/streamout_blocks\\/R2020a\"],\"version\":\"1.0\"}"  VisualizationBindings="{\"xyplotplugin\":{\"info\":[{\"series\":[],\"subplotID\":1}]}}"  CompatibilityTag=XY
  Thetam : Outport
  Wm : Outport  Port=2
  wires:
  Tld [N.m]/1 -> Gain4/1
  Gain3/1 -> Trigonometric Function/1  "Thetal[rad]"
  Tm[N.m]/1 -> XY Graph/2, Sum1/2  "Tm[N.m]"
  Integrator/1 -> XY Graph/1, Wm/1, Gain1/1, Integrator1/1  "Wm[rad/s]"
  Integrator1/1 -> Thetam/1, Gain3/1  "Thetam[rad]"
  Trigonometric Function/1 -> Gain2/1
  Gain1/1 -> TorqueFriccion/1, Sum1/3
  Gain/1 -> Integrator/1  "dWm/dt[rad/s^2]"
  Sum1/1 -> TorqueEq/1, Gain/1
  Gain4/1 -> Sum2/1
  Gain2/1 -> Sum2/2
  Sum2/1 -> Perturbacion TL/1, Sum1/1

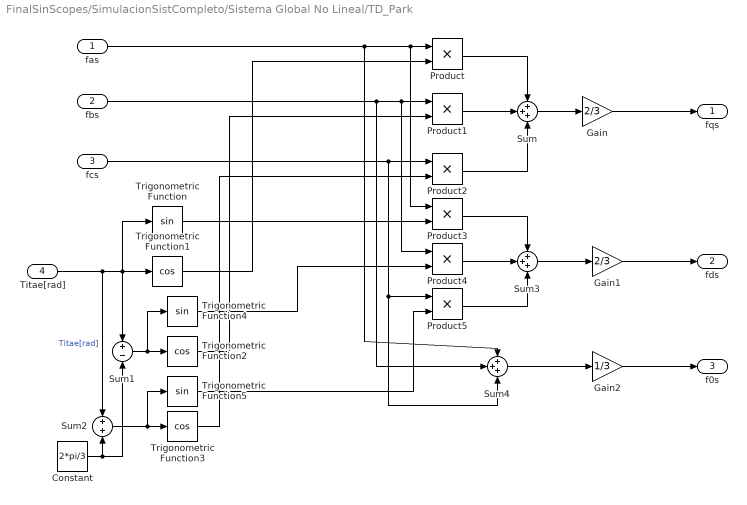
== system FinalSinScopes/SimulacionSistCompleto/Sistema Global No Lineal/TD_Park ==
  fas : Inport
  fbs : Inport  Port=2
  fcs : Inport  Port=3
  Titae[rad] : Inport  Port=4
  Constant : Constant  Value=2*pi/3
  Gain : Gain  Gain=2/3
  Gain1 : Gain  Gain=2/3
  Gain2 : Gain  Gain=1/3
  Product{,1..5} (6 alike) : Product
  Sum : Sum  Inputs=+++
  Sum1 : Sum  Inputs=+-
  Sum2 : Sum
  Sum3 : Sum  Inputs=+++
  Sum4 : Sum  Inputs=+++
  Trigonometric Function : Trigonometry
  Trigonometric Function1 : Trigonometry  Operator=cos
  Trigonometric Function2 : Trigonometry  Operator=cos
  Trigonometric Function3 : Trigonometry  Operator=cos
  Trigonometric Function4 : Trigonometry
  Trigonometric Function5 : Trigonometry
  fqs : Outport
  fds : Outport  Port=2
  f0s : Outport  Port=3
  wires:
  fas/1 -> Sum4/1, Product3/1, Product/1
  Trigonometric Function3/1 -> Product2/2
  Sum1/1 -> Trigonometric Function4/1, Trigonometric Function2/1
  Constant/1 -> Sum2/2, Sum1/2
  Trigonometric Function1/1 -> Product/2
  fcs/1 -> Product5/1, Sum4/3, Product2/1
  Product5/1 -> Sum3/3
  Product/1 -> Sum/1
  Product3/1 -> Sum3/1
  Product1/1 -> Sum/2
  Trigonometric Function/1 -> Product3/2
  Sum2/1 -> Trigonometric Function5/1, Trigonometric Function3/1
  Trigonometric Function5/1 -> Product5/2
  Sum4/1 -> Gain2/1
  fbs/1 -> Sum4/2, Product4/1, Product1/1
  Product2/1 -> Sum/3
  Gain/1 -> fqs/1
  Trigonometric Function4/1 -> Product4/2
  Product4/1 -> Sum3/2
  Trigonometric Function2/1 -> Product1/2
  Gain2/1 -> f0s/1
  Sum/1 -> Gain/1
  Gain1/1 -> fds/1
  Sum3/1 -> Gain1/1
  Titae[rad]/1 -> Sum2/1, Trigonometric Function/1, Sum1/1, Trigonometric Function1/1  "Titae[rad]"

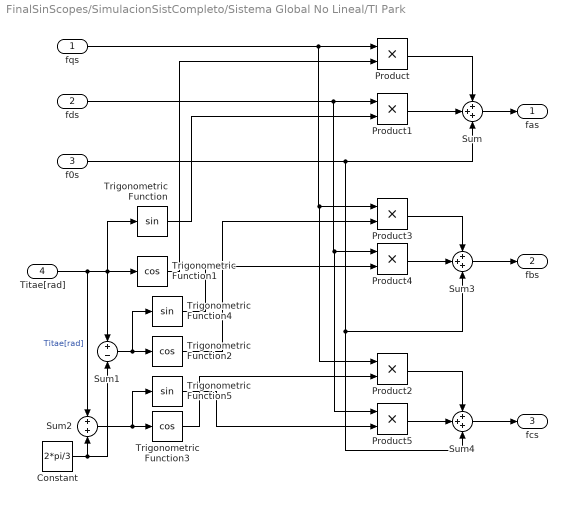
== system FinalSinScopes/SimulacionSistCompleto/Sistema Global No Lineal/TI Park ==
  fqs : Inport
  fds : Inport  Port=2
  f0s : Inport  Port=3
  Titae[rad] : Inport  Port=4
  Constant : Constant  Value=2*pi/3
  Product{,1..5} (6 alike) : Product
  Sum : Sum  Inputs=+++
  Sum1 : Sum  Inputs=+-
  Sum2 : Sum
  Sum3 : Sum  Inputs=+++
  Sum4 : Sum  Inputs=+++
  Trigonometric Function : Trigonometry
  Trigonometric Function1 : Trigonometry  Operator=cos
  Trigonometric Function2 : Trigonometry  Operator=cos
  Trigonometric Function3 : Trigonometry  Operator=cos
  Trigonometric Function4 : Trigonometry
  Trigonometric Function5 : Trigonometry
  fas : Outport
  fbs : Outport  Port=2
  fcs : Outport  Port=3
  wires:
  Constant/1 -> Sum2/2, Sum1/2
  Product1/1 -> Sum/2
  Trigonometric Function2/1 -> Product3/2
  Trigonometric Function5/1 -> Product5/2
  fds/1 -> Product1/1, Product5/1, Product4/1
  f0s/1 -> Sum/3, Sum3/3, Sum4/3
  Product3/1 -> Sum3/1
  fqs/1 -> Product/1, Product2/1, Product3/1
  Product2/1 -> Sum4/1
  Trigonometric Function1/1 -> Product/2
  Product/1 -> Sum/1
  Sum2/1 -> Trigonometric Function5/1, Trigonometric Function3/1
  Sum1/1 -> Trigonometric Function4/1, Trigonometric Function2/1
  Trigonometric Function/1 -> Product1/2
  Product4/1 -> Sum3/2
  Sum/1 -> fas/1
  Trigonometric Function3/1 -> Product2/2
  Product5/1 -> Sum4/2
  Trigonometric Function4/1 -> Product4/2
  Sum3/1 -> fbs/1
  Sum4/1 -> fcs/1
  Titae[rad]/1 -> Sum2/1, Trigonometric Function/1, Sum1/1, Trigonometric Function1/1  "Titae[rad]"

== matlab function FinalSinScopes/Consigna Suavizada ==
  data: t input; y output
function y = trapecio_periodico(t)
    % Parámetros
    T = 15;              % Periodo total
    ramp_time = 0.5;     % Duración de la rampa (en segundos)
    amplitude = 2 * pi / 5; % Amplitud del trapecio

    % Calcular el tiempo dentro del período
    t_mod = mod(t, T);

    % Inicializar salida
    y = 0;

    % Fase 1: Primer trapecio (0 <= t_mod < 5)
    if t_mod >= 0 && t_mod < 5
        if t_mod < ramp_time
            % Rampa ascendente (inicio)
            y = amplitude * (t_mod / ramp_time);
        elseif t_mod >= ramp_time && t_mod <= (5 - ramp_time)
            % Parte constante (plataforma)
            y = amplitude;
        elseif t_mod > (5 - ramp_time) && t_mod <= 5
            % Rampa descendente (fin)
            y = amplitude * (1 - (t_mod - (5 - ramp_time)) / ramp_time);
        end
    end

    % Fase 2: Segundo trapecio (-2*pi/5) (10 <= t_mod < 15)
    if t_mod >= 10 && t_mod < 15
        if t_mod < (10 + ramp_time)
            % Rampa descendente (inicio)
            y = -amplitude * ((t_mod - 10) / ramp_time);
        elseif t_mod >= (10 + ramp_time) && t_mod <= (15 - ramp_time)
            % Parte constante (plataforma)
            y = -amplitude;
        elseif t_mod > (15 - ramp_time) && t_mod < 15
            % Rampa ascendente (fin)
            y = -amplitude * (1 - (t_mod - (15 - ramp_time)) / ramp_time);
        end
    end
end
